simulink model "pwm_Test"  (R2018b)
settings: Solver=FixedStepAuto  StartTime=0.0  StopTime=inf  FixedStep=.001  RelTol=1e-3  EnableMultiTasking=on
settings Model: SimulationMode=external  Creator=dskaputa  LastModifiedBy=dskaputa
settings SolverCC: PositivePriorityOrder=on
settings OptimizationCC: PassReuseOutputArgsAs=Individual arguments  MaxStackSize=64
settings DebuggingCC: ParameterTunabilityLossMsg=error
settings HardwareCC: ProdBitPerPointer=32  ProdBitPerSizeT=32  ProdBitPerPtrDiffT=32  ProdLargestAtomicInteger=Long  ProdLargestAtomicFloat=Double  ProdWordSize=32  ProdHWDeviceType=ARM Compatible->ARM Cortex
settings SFSimCC: SimUseLocalCustomCode=off  MATLABDynamicMemAlloc=off
settings RTWCC: SystemTargetFile=ert.tlc  HardwareBoard=Xilinx Zynq-7000 based board  TLCOptions="-aInlineSetEventsForThisBaseRateFcn=TLC_FALSE -aSuppressMultiTaskScheduler=TLC_FALSE  -aRateBasedStepFcn=0"  TemplateMakefile=ert_default_tmf  GenerateReport=on  RTWUseLocalCustomCode=off  Toolchain=Linaro AArch32 Linux v6.3.1  IncludeHyperlinkInReport=on  LaunchReport=on  GenerateTraceInfo=on  GenerateTraceReport=on  GenerateTraceReportSl=on  GenerateTraceReportSf=on  GenerateTraceReportEml=on
settings CodeAppCC: ForceParamTrailComments=on  IgnoreCustomStorageClasses=off  OperatorAnnotations=on  SimulinkDataObjDesc=on  SFDataObjDesc=on  MATLABFcnDesc=on  InsertBlockDesc=on  StateflowObjectComments=on  MATLABSourceComments=on
settings ERTTargetCC: SupportNonInlinedSFcns=on

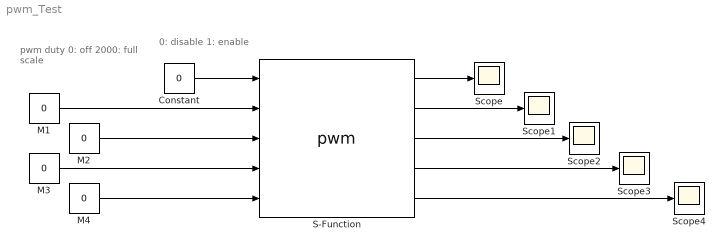
== system pwm_Test ==
  note: pwm duty
      | 0: off
      | 2000: full scale
  note: 0: disable
      | 1: enable
  Constant : Constant  Value=0  SampleTime=-1
  M{1..4} (4 alike) : Constant  Value=0  SampleTime=-1
  S-Function : S-Function  FunctionName=pwm  SFunctionDeploymentMode=off  EnableBusSupport=off
      mask Display: image('pwm.jpg');
  Scope{,1..4} (5 alike) : Scope
  wires:
  Constant/1 -> S-Function/1
  M1/1 -> S-Function/2
  S-Function/1 -> Scope/1
  S-Function/2 -> Scope1/1
  S-Function/3 -> Scope2/1
  S-Function/4 -> Scope3/1
  S-Function/5 -> Scope4/1
  M2/1 -> S-Function/3
  M3/1 -> S-Function/4
  M4/1 -> S-Function/5
